simulink model "LUPAold"  (R2025b)
settings: Solver=FixedStepAuto  StartTime=0.0  StopTime=inf  FixedStep=Ts  RelTol=1e-3
PreLoadFcn:
  | addpath(genpath('utils'))
model workspace (MAT data in the model file):
  Sig = Simulink.Signal
  Sig.Dimensions = -1
  Sig.DimensionsMode = 'auto'
  Sig.Complexity = 'auto'
  Sig.SampleTime = -1
  Sig.SamplingMode = 'auto'
  Sig.DataType = 'auto'
values from neighbouring files (symbols this model uses):
  C = 258.803991051052    (= 258.803991051)    [AOE_constants.m]
  ExcelGains = table2array(ExcelGains)    [initLUPA.m]
  gainTstep = wavePeriod*10    (= 22.5)    [initLUPA.m]
  Kt = 7.86    [initLUPA.m]
  rampTime = 20    [initLUPA.m]
  sprocketPitchRadius = 0.101854    [initLUPA.m]
  Ts = 0.001    [initLUPA.m]
undefined symbols (not defined in the file or in its folder): drawWire_m, drawWire_mpers, eCATstate, linearPower_W, netForce_N, opState, pos_filt_rad, tet, vel_filt_radpers
libraries: slrealtimeethercatlib x26, slrealtimeloglib x12, simulink x6, dspfdesign x6, slrealtimeutilitieslib x4, dspstat3 x3, eeGeneralControl x3, slrealtimeptplib x1, slrealtimetgmanagement x1
settings Model: SimulationMode=external  ExtModeEnableFloating=off  Creator=HWRL user  LastModifiedBy=bosmab
settings SolverCC: ConcurrentTasks=on  PositivePriorityOrder=on
settings DataIOCC: ExternalInput=ds  LoadExternalInput=on
settings OptimizationCC: BlockReduction=off  OptimizeBlockIOStorage=off  ReuseModelBlockBuffer=off
settings DebuggingCC: TasksWithSamePriorityMsg=none  ParameterOverflowMsg=warning  ParameterPrecisionLossMsg=none  UnconnectedInputMsg=warning  UnconnectedOutputMsg=warning  UnconnectedLineMsg=warning
settings HardwareCC: ProdBitPerLong=64.0  ProdLongLongMode=on  ProdHWDeviceType=Intel->x86-64 (Linux 64)
settings ModelReferenceCC: EnableRefExpFcnMdlSchedulingChecks=on
settings SFSimCC: SimTargetLang=C++  SimDLTargetLibrary=mkl-dnn
settings RTWCC: SystemTargetFile=speedgoat.tlc  TemplateMakefile=slrealtime_default_tmf  RTWVerbose=off  Toolchain=Simulink Real-Time Toolchain  BuildConfiguration=Faster Runs  CodeExecutionProfiling=on  TargetLang=C++  GPUComputeCapability=3.5  DLArmComputeVersion=19.05  Description=Speedgoat Real-Time Target Machine
settings SimulinkRealTimeTargetCC: SLRTFileLogMaxRuns=1.0  ExtModeMaxTrigDuration=10.0  ExtModeStaticAllocSize=1000000.0  ExtModeTransport=0.0  MultiwordLength=2048.0  DynamicStringBufferSize=256.0  PreserveMATLABNamespacesInGeneratedCode=on  SubcomponentCodeInterfacePackaging=Reusable function  InstructionSetFMA=off  LogToMDFFile=off

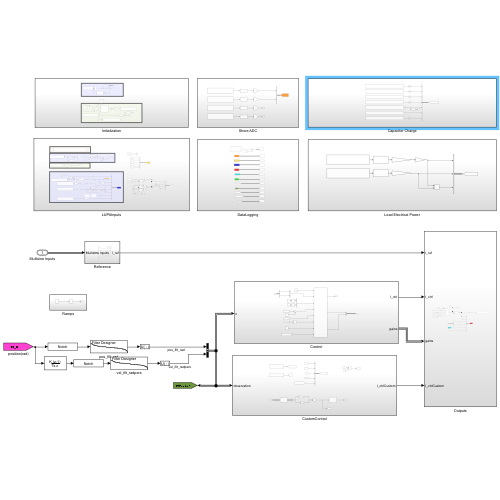
[thumbnail: Simulink's stored preview of the top-level diagram]
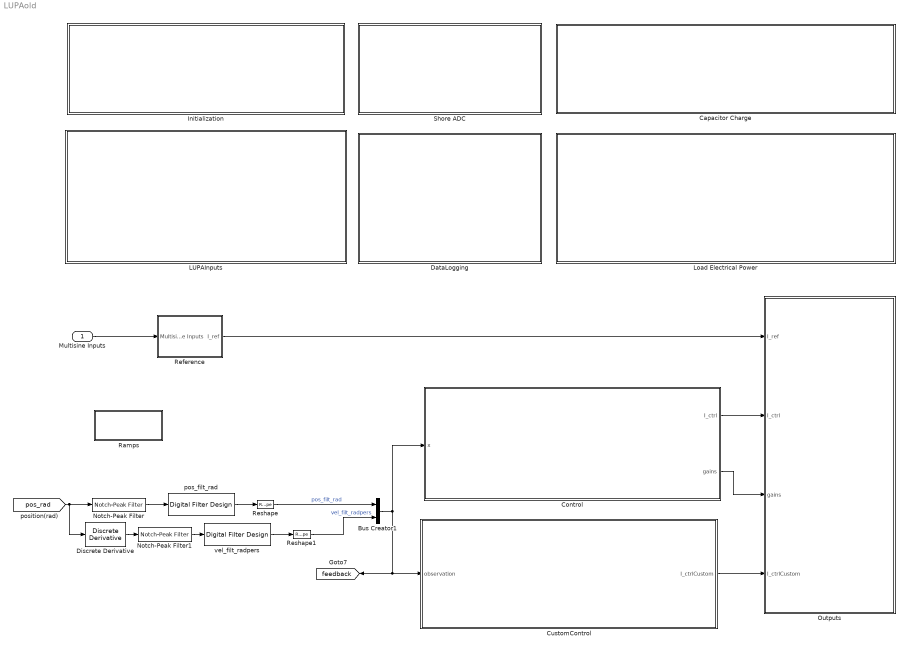
== system LUPAold ==
  Multisine Inputs : Inport  OutDataTypeStr=Bus: refSigs
  Bus Creator1 : BusCreator  Inputs=pos_filt_rad,vel_filt_radpers
  Capacitor Charge : Subsystem
  Control : Subsystem
  CustomControl : Subsystem
  DataLogging : Subsystem
  Discrete Derivative : simulink/Discrete/Discrete Derivative  gainval=1.0  ICPrevScaledInput=0.0  OutMin=[]  OutMax=[]  OutDataType=fixdt(1, 16)  OutScaling=2^-10  DoSatur=off
  Initialization : Subsystem
  LUPAInputs : Subsystem
  Load Electrical Power : Subsystem
  Notch-Peak Filter : dspfdesign/Notch-Peak Filter  Specification=Bandwidth and center frequency  BandwidthPort=off  Bandwidth=10  QualityFactorPort=off  QualityFactor=5  CenterFrequencyPort=off  CenterFrequency=50  BandwidthCoefficientPort=off  BandwidthCoefficient=0.72654  CenterFrequencyCoefficientPort=off  CenterFrequencyCoefficient=0  Output=Notch  SampleRateMode=Specify on dialog  SampleRate=1000  SimulateUsing=Code generation
  Notch-Peak Filter1 : dspfdesign/Notch-Peak Filter  Specification=Bandwidth and center frequency  BandwidthPort=off  Bandwidth=10  QualityFactorPort=off  QualityFactor=5  CenterFrequencyPort=off  CenterFrequency=50  BandwidthCoefficientPort=off  BandwidthCoefficient=0.72654  CenterFrequencyCoefficientPort=off  CenterFrequencyCoefficient=0  Output=Notch  SampleRateMode=Specify on dialog  SampleRate=1000  SimulateUsing=Code generation
  Outputs : Subsystem
  Ramps : Subsystem
  Reference : Subsystem
  Reshape : Reshape
  Reshape1 : Reshape
  Shore ADC : Subsystem
  pos_filt_rad : dspfdesign/Digital Filter Design  mwdsp_browser_bugfix_var=off
  vel_filt_radpers : dspfdesign/Digital Filter Design  mwdsp_browser_bugfix_var=off
  tag scope: feedback=global
  wires:
  Control/1(I_ctrl) -> Outputs/2(I_ctrl)
  Bus Creator1/1 -> Control/1(x), [feedback], CustomControl/1(observation)
  [pos_rad] -> Discrete Derivative/1, Notch-Peak Filter/1
  Control/2(gains) -> Outputs/3(gains)
  CustomControl/1(I_ctrlCustom) -> Outputs/4(I_ctrlCustom)
  Reference/1(I_ref) -> Outputs/1(I_ref)
  Multisine Inputs/1 -> Reference/1(Multisine Inputs)
  Notch-Peak Filter/1 -> pos_filt_rad/1
  Notch-Peak Filter1/1 -> vel_filt_radpers/1
  Discrete Derivative/1 -> Notch-Peak Filter1/1
  pos_filt_rad/1 -> Reshape/1
  vel_filt_radpers/1 -> Reshape1/1
  Reshape/1 -> Bus Creator1/1  "pos_filt_rad"
  Reshape1/1 -> Bus Creator1/2  "vel_filt_radpers"

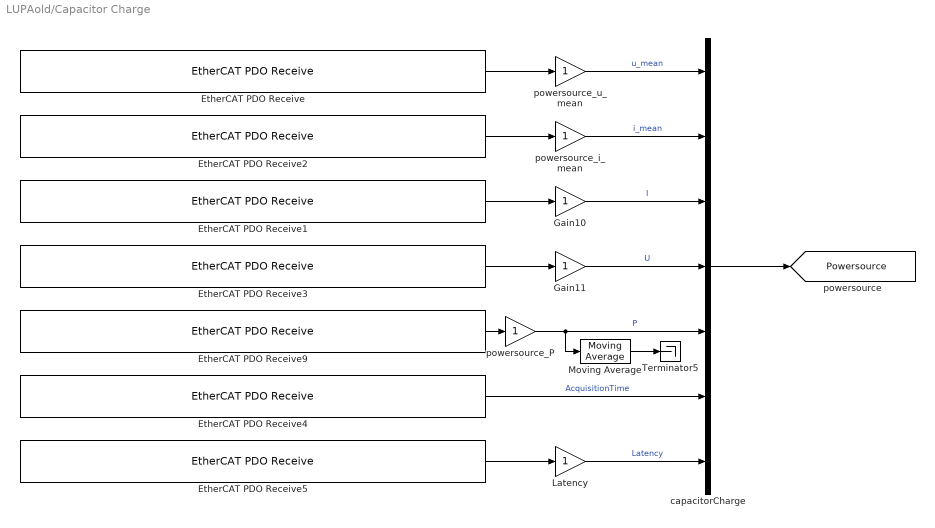
== system LUPAold/Capacitor Charge ==
  EtherCAT PDO Receive : slrealtimeethercatlib/EtherCAT PDO Receive  Priority=2  sig_name=Box 1 (GEN Series DAQ System).Powersource.out.u_mean.Powersource.out.u_mean_V  sig_offset=2648  sig_type=single  type_size=32  sig_dim=1  device_id=0  sample_time=0.001000
  EtherCAT PDO Receive1 : slrealtimeethercatlib/EtherCAT PDO Receive  Priority=2  sig_name=Box 1 (GEN Series DAQ System).Powersource.out.I.Powersource.out.I_V  sig_offset=2528  sig_type=single  type_size=32  sig_dim=1  device_id=0  sample_time=0.001000
  EtherCAT PDO Receive2 : slrealtimeethercatlib/EtherCAT PDO Receive  Priority=2  sig_name=Box 1 (GEN Series DAQ System).Powersource.out.i_mean.Powersource.out.i_mean_V  sig_offset=2608  sig_type=single  type_size=32  sig_dim=1  device_id=0  sample_time=0.001000
  EtherCAT PDO Receive3 : slrealtimeethercatlib/EtherCAT PDO Receive  Priority=2  sig_name=Box 1 (GEN Series DAQ System).Powersource.out.U.Powersource.out.U_V  sig_offset=2568  sig_type=single  type_size=32  sig_dim=1  device_id=0  sample_time=0.001000
  EtherCAT PDO Receive4 : slrealtimeethercatlib/EtherCAT PDO Receive  Priority=2  sig_name=Box 1 (GEN Series DAQ System).AcquisitionTime.AcquisitionTime_V  sig_offset=2296  sig_type=double  type_size=64  sig_dim=1  device_id=0  sample_time=0.001000
  EtherCAT PDO Receive5 : slrealtimeethercatlib/EtherCAT PDO Receive  Priority=2  sig_name=Box 1 (GEN Series DAQ System).Latency.Latency_V  sig_offset=2368  sig_type=single  type_size=32  sig_dim=1  device_id=0  sample_time=0.001000
  EtherCAT PDO Receive9 : slrealtimeethercatlib/EtherCAT PDO Receive  Priority=2  sig_name=Box 1 (GEN Series DAQ System).Powersource.out.P.Powersource.out.P_V  sig_offset=2688  sig_type=single  type_size=32  sig_dim=1  device_id=0  sample_time=0.001000
  Gain10 : Gain  OutDataTypeStr=double
  Gain11 : Gain  OutDataTypeStr=double
  Latency : Gain  OutDataTypeStr=double
  Moving Average : dspstat3/Moving Average  Method=Sliding window  ForgettingFactorPort=off  SpecifyWindowLength=on  WindowLength=10000  OverlapLength=9000  AllowArbitraryInputLength=on  ForgettingFactor=0.9  SimulateUsing=Code generation
  Terminator5 : Terminator
  capacitorCharge : BusCreator  Inputs=7
  powersource_P : Gain  OutDataTypeStr=double
  powersource_i_mean : Gain  OutDataTypeStr=double
  powersource_u_mean : Gain  OutDataTypeStr=double
  tag scope: Powersource=global
  wires:
  powersource_u_mean/1 -> capacitorCharge/1  "u_mean"
  powersource_i_mean/1 -> capacitorCharge/2  "i_mean"
  capacitorCharge/1 -> [Powersource]
  Gain10/1 -> capacitorCharge/3  "I"
  Gain11/1 -> capacitorCharge/4  "U"
  EtherCAT PDO Receive/1 -> powersource_u_mean/1
  EtherCAT PDO Receive2/1 -> powersource_i_mean/1
  EtherCAT PDO Receive1/1 -> Gain10/1
  EtherCAT PDO Receive3/1 -> Gain11/1
  EtherCAT PDO Receive9/1 -> powersource_P/1
  powersource_P/1 -> Moving Average/1, capacitorCharge/5  "P"
  EtherCAT PDO Receive4/1 -> capacitorCharge/6  "AcquisitionTime"
  EtherCAT PDO Receive5/1 -> Latency/1
  Latency/1 -> capacitorCharge/7  "Latency"
  Moving Average/1 -> Terminator5/1

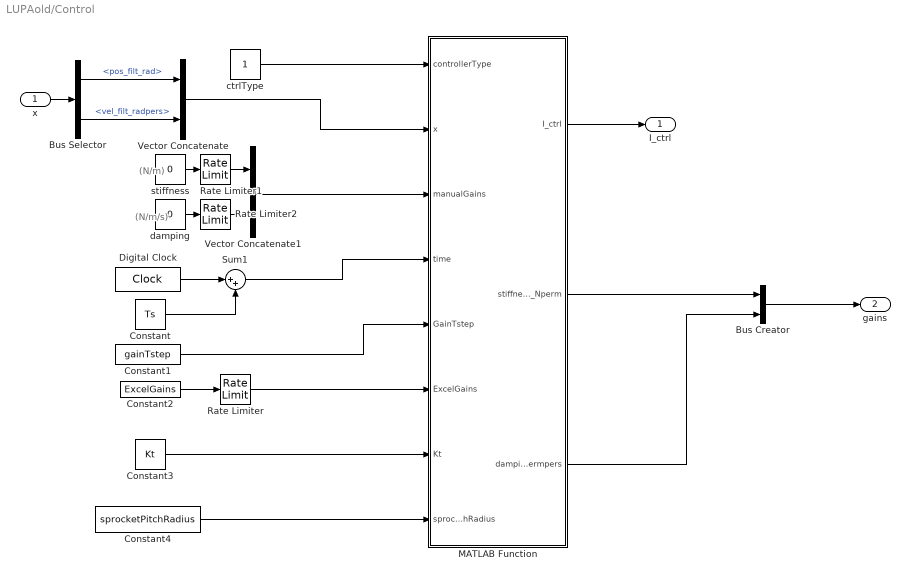
== system LUPAold/Control ==
  note: (N/m/s)
  note: (N/m)
  x : Inport
  Bus Creator : BusCreator  Inputs=2
  Bus Selector : BusSelector  OutputSignals=pos_filt_rad,vel_filt_radpers
  Constant : Constant  Value=Ts
  Constant1 : Constant  Value=gainTstep
  Constant2 : Constant  Value=ExcelGains  VectorParams1D=off
  Constant3 : Constant  Value=Kt
  Constant4 : Constant  Value=sprocketPitchRadius
  Digital Clock : DigitalClock  SampleTime=Ts
  MATLAB Function : MATLAB Function  TreatAsAtomicUnit=on
  Rate Limiter : RateLimiter  RisingSlewLimit=200  FallingSlewLimit=-200  SampleTimeMode=inherited
  Rate Limiter1 : RateLimiter  RisingSlewLimit=200  FallingSlewLimit=-200  SampleTimeMode=inherited
  Rate Limiter2 : RateLimiter  RisingSlewLimit=200  FallingSlewLimit=-200  SampleTimeMode=inherited
  Sum1 : Sum  Inputs=|++
  Vector Concatenate : Concatenate  Mode=Multidimensional array
  Vector Concatenate1 : Concatenate  Mode=Multidimensional array
  ctrlType : Constant
  damping : Constant  Value=0
  stiffness : Constant  Value=0
  I_ctrl : Outport
  gains : Outport  Port=2
  wires:
  stiffness/1 -> Rate Limiter1/1
  Constant1/1 -> MATLAB Function/5(GainTstep)
  Constant/1 -> Sum1/2
  Vector Concatenate1/1 -> MATLAB Function/3(manualGains)
  Digital Clock/1 -> Sum1/1
  x/1 -> Bus Selector/1
  Sum1/1 -> MATLAB Function/4(time)
  Constant4/1 -> MATLAB Function/8(sprocketPitchRadius)
  damping/1 -> Rate Limiter2/1
  Vector Concatenate/1 -> MATLAB Function/2(x)
  ctrlType/1 -> MATLAB Function/1(controllerType)
  Constant3/1 -> MATLAB Function/7(Kt)
  Constant2/1 -> Rate Limiter/1
  Bus Selector/1 -> Vector Concatenate/1  "<pos_filt_rad>"
  Bus Selector/2 -> Vector Concatenate/2  "<vel_filt_radpers>"
  MATLAB Function/1(I_ctrl) -> I_ctrl/1
  MATLAB Function/2(stiffness_Nperm) -> Bus Creator/1
  MATLAB Function/3(damping_Npermpers) -> Bus Creator/2
  Bus Creator/1 -> gains/1
  Rate Limiter/1 -> MATLAB Function/6(ExcelGains)
  Rate Limiter1/1 -> Vector Concatenate1/1
  Rate Limiter2/1 -> Vector Concatenate1/2

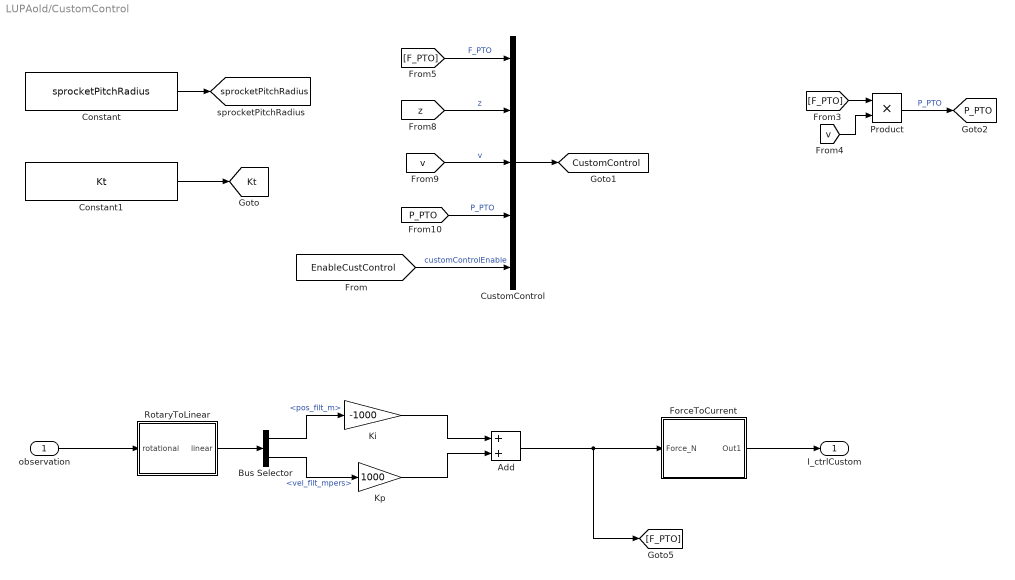
== system LUPAold/CustomControl ==
  observation : Inport
  Add : Sum
  Bus Selector : BusSelector  OutputSignals=pos_filt_m,vel_filt_mpers
  Constant : Constant  Value=sprocketPitchRadius
  Constant1 : Constant  Value=Kt
  CustomControl : BusCreator  Inputs=5
  ForceToCurrent : Subsystem
  Ki : Gain  Gain=-1000
  Kp : Gain  Gain=1000
  Product : Product
  RotaryToLinear : Subsystem
  I_ctrlCustom : Outport
  tag scope: CustomControl=global, Kt=global, P_PTO=global, sprocketPitchRadius=global
  wires:
  Constant/1 -> [sprocketPitchRadius]
  Constant1/1 -> [Kt]
  ForceToCurrent/1(Out1) -> I_ctrlCustom/1
  [F_PTO] -> Product/1
  [v] -> Product/2
  Product/1 -> [P_PTO]  "P_PTO"
  observation/1 -> RotaryToLinear/1(rotational)
  CustomControl/1 -> [CustomControl]
  [F_PTO] -> CustomControl/1  "F_PTO"
  [z] -> CustomControl/2  "z"
  [v] -> CustomControl/3  "v"
  [P_PTO] -> CustomControl/4  "P_PTO"
  RotaryToLinear/1(linear) -> Bus Selector/1
  Bus Selector/1 -> Ki/1  "<pos_filt_m>"
  Bus Selector/2 -> Kp/1  "<vel_filt_mpers>"
  Ki/1 -> Add/1
  Kp/1 -> Add/2
  Add/1 -> [F_PTO], ForceToCurrent/1(Force_N)
  [EnableCustControl] -> CustomControl/5  "customControlEnable"

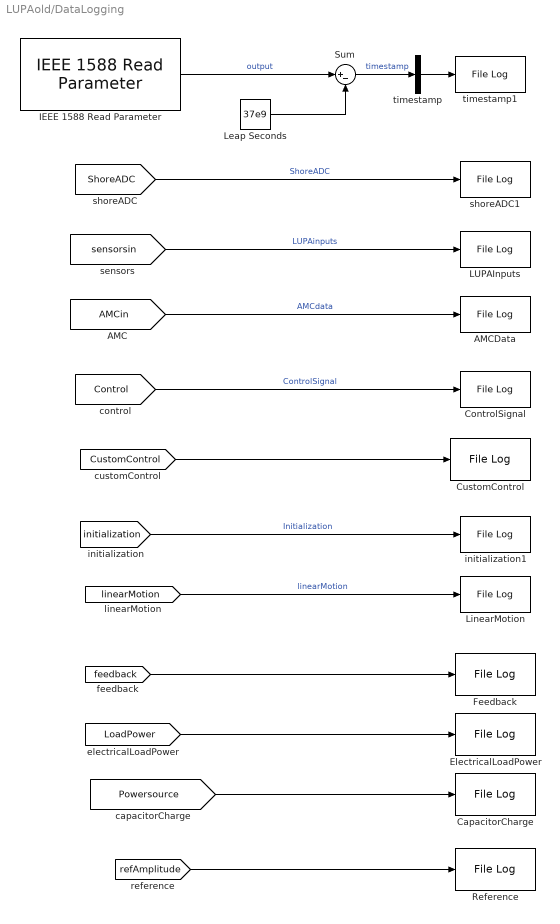
== system LUPAold/DataLogging ==
  AMCData : slrealtimeloglib/File Log  decimation=decimationLog  inputProcessing=Elements as channels (sample based)
  CapacitorCharge : slrealtimeloglib/File Log  decimation=1  inputProcessing=Elements as channels (sample based)
  ControlSignal : slrealtimeloglib/File Log  decimation=decimationLog  inputProcessing=Elements as channels (sample based)
  CustomControl : slrealtimeloglib/File Log  decimation=decimationLog  inputProcessing=Elements as channels (sample based)
  ElectricalLoadPower : slrealtimeloglib/File Log  decimation=1  inputProcessing=Elements as channels (sample based)
  Feedback : slrealtimeloglib/File Log  decimation=1  inputProcessing=Elements as channels (sample based)
  IEEE 1588 Read Parameter : slrealtimeptplib/IEEE 1588 Read Parameter  Priority=1  ID=1  param=1. System time (nanosecond)  sample_time=Ts
  LUPAInputs : slrealtimeloglib/File Log  decimation=decimationLog  inputProcessing=Elements as channels (sample based)
  Leap Seconds : Constant  Value=37e9  OutDataTypeStr=double
  LinearMotion : slrealtimeloglib/File Log  decimation=decimationLog  inputProcessing=Elements as channels (sample based)
  Reference : slrealtimeloglib/File Log  decimation=1  inputProcessing=Elements as channels (sample based)
  Sum : Sum  Inputs=|+-
  initialization1 : slrealtimeloglib/File Log  decimation=decimationLog  inputProcessing=Elements as channels (sample based)
  shoreADC1 : slrealtimeloglib/File Log  decimation=decimationLog  inputProcessing=Elements as channels (sample based)
  timestamp : BusCreator  Inputs=timestamp
  timestamp1 : slrealtimeloglib/File Log  decimation=decimationLog  inputProcessing=Elements as channels (sample based)
  wires:
  [AMCin] -> AMCData/1  "AMCdata"
  [Control] -> ControlSignal/1  "ControlSignal"
  IEEE 1588 Read Parameter/1 -> Sum/1  "output"
  Sum/1 -> timestamp/1  "timestamp"
  timestamp/1 -> timestamp1/1
  Leap Seconds/1 -> Sum/2
  [initialization] -> initialization1/1  "Initialization"
  [sensorsin] -> LUPAInputs/1  "LUPAinputs"
  [ShoreADC] -> shoreADC1/1  "ShoreADC"
  [linearMotion] -> LinearMotion/1  "linearMotion"
  [feedback] -> Feedback/1
  [CustomControl] -> CustomControl/1
  [LoadPower] -> ElectricalLoadPower/1
  [Powersource] -> CapacitorCharge/1
  [refAmplitude] -> Reference/1

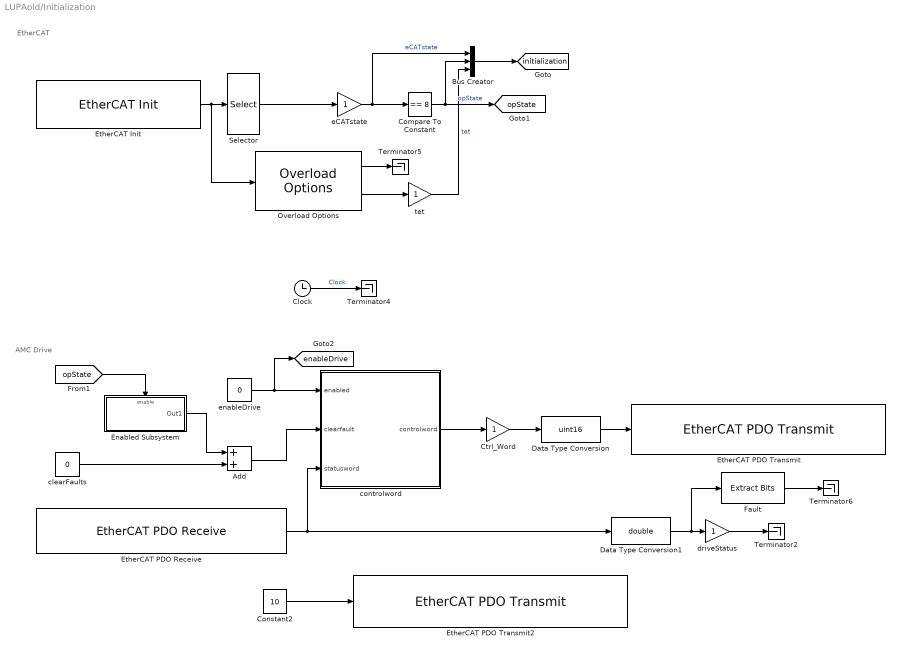
== system LUPAold/Initialization ==
  note: AMC Drive
  note: EtherCAT
  Add : Sum
  Bus Creator : BusCreator  Inputs=eCATstate,opState,tet
  Clock : Clock
  Compare To Constant : simulink/Logic and Bit Operations/Compare To Constant  relop===  const=8  OutDataTypeStr=boolean
  Constant2 : Constant  Value=10  OutDataTypeStr=uint16
  Ctrl_Word : Gain
  Data Type Conversion : DataTypeConversion  OutDataTypeStr=uint16  SaturateOnIntegerOverflow=off  RndMeth=Floor
  Data Type Conversion1 : DataTypeConversion  OutDataTypeStr=double  SaturateOnIntegerOverflow=off  RndMeth=Floor
  Enabled Subsystem : Subsystem  TreatAsAtomicUnit=on
  EtherCAT Init : slrealtimeethercatlib/EtherCAT Init  Priority=0  config_file=C:\Software\LUPA\Simulink\EtherCAT\LUPAxml.xml  device_id=0  portnum=1  initstate=2  dctuning=0  enaDebug=0  logFile='c:\dbglog.txt'  sample_time=0.001000  DCMode=2
  EtherCAT PDO Receive : slrealtimeethercatlib/EtherCAT PDO Receive  Priority=2  sig_name=Drive 7 (AMC - DPE X2.1).PDO data from Slave.Status Word  sig_offset=576  sig_type=uint16  type_size=16  sig_dim=1  device_id=0  sample_time=0.001000
  EtherCAT PDO Transmit : slrealtimeethercatlib/EtherCAT PDO Transmit  Priority=3  sig_name=Drive 7 (AMC - DPE X2.1).PDO data to Slave.Control Word  sig_offset=576  sig_type=uint16  type_size=16  sig_dim=1  device_id=0  sample_time=0.001000
  EtherCAT PDO Transmit2 : slrealtimeethercatlib/EtherCAT PDO Transmit  Priority=3  sig_name=Drive 7 (AMC - DPE X2.1).PDO data to Slave.Modes Of Operation  sig_offset=688  sig_type=uint16  type_size=16  sig_dim=1  device_id=0  sample_time=0.001000
  Fault : simulink/Logic and Bit Operations/Extract Bits  bitsToExtract=Range of bits  numBits=8  bitIdxRange=[3]  outScalingMode=Preserve fixed-point scaling
  Overload Options : slrealtimetgmanagement/Overload Options  startupDur=1  startupDurSrc=Tunable Parameter  maxOverload=0  maxOverloadSrc=Tunable Parameter  TETFlag=on
  Selector : Selector  InputPortWidth=6  IndexOptions=Index vector (dialog)  Indices=2  OutputSizes=1
  Terminator{2,4..6} (4 alike) : Terminator
  clearFaults : Constant  Value=0
  controlword : MATLAB Function  TreatAsAtomicUnit=on
  driveStatus : Gain
  eCATstate : Gain  OutDataTypeStr=double
  enableDrive : Constant  Value=0
  tet : Gain  OutDataTypeStr=double
  tag scope: enableDrive=global, initialization=global, opState=global
  wires:
  EtherCAT Init/1 -> Overload Options/1, Selector/1
  Selector/1 -> eCATstate/1
  Compare To Constant/1 -> [opState], Bus Creator/2  "opState"
  EtherCAT PDO Receive/1 -> Data Type Conversion1/1, controlword/3(statusword)
  Constant2/1 -> EtherCAT PDO Transmit2/1
  Data Type Conversion1/1 -> Fault/1, driveStatus/1
  controlword/1(controlword) -> Ctrl_Word/1
  Data Type Conversion/1 -> EtherCAT PDO Transmit/1
  driveStatus/1 -> Terminator2/1
  Ctrl_Word/1 -> Data Type Conversion/1
  enableDrive/1 -> [enableDrive], controlword/1(enabled)
  eCATstate/1 -> Bus Creator/1, Compare To Constant/1  "eCATstate"
  Clock/1 -> Terminator4/1  "Clock"
  Bus Creator/1 -> [initialization]
  Overload Options/2 -> tet/1
  tet/1 -> Bus Creator/3  "tet"
  Overload Options/1 -> Terminator5/1
  Fault/1 -> Terminator6/1
  Enabled Subsystem/1(Out1) -> Add/1
  [opState] -> Enabled Subsystem/Enable
  Add/1 -> controlword/2(clearfault)
  clearFaults/1 -> Add/2

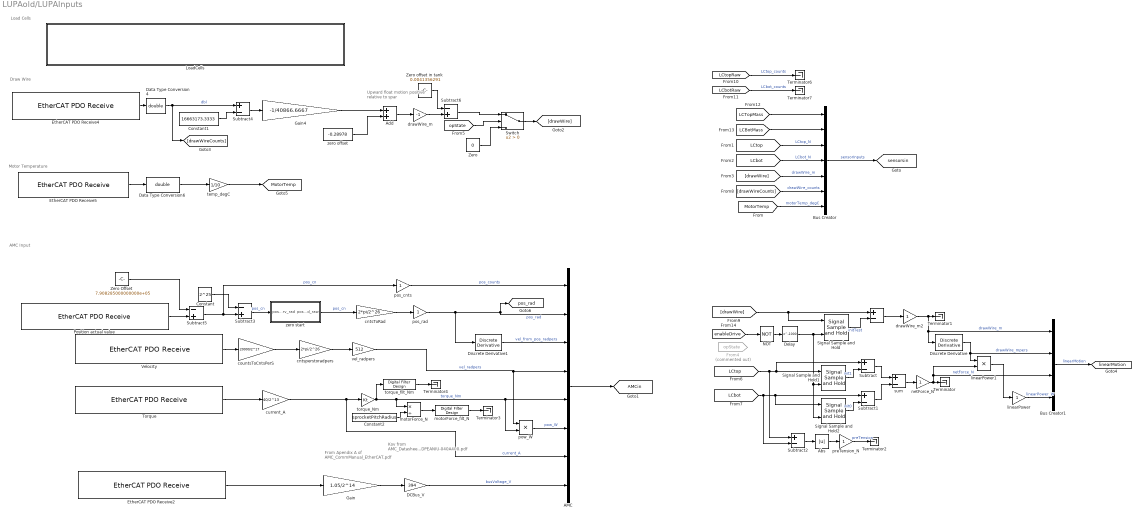
== system LUPAold/LUPAInputs ==
  note: Load Cells
  note: Upward float motion
      | positive relative to spar
  note: Draw Wire
  note: Motor Temperature
  note: From Apendix A of AMC_CommManual_EtherCAT.pdf
  note: AMC Input
  note: Kov from AMC_Datasheet_DPEANIU-040A400.pdf
  " " : Sum  Inputs=+-
  AMC : BusCreator  Inputs=8
  Abs : Abs  SaturateOnIntegerOverflow=off
  Add : Sum
  Bus Creator : BusCreator  Inputs=7
  Bus Creator1 : BusCreator  Inputs=drawWire_m,drawWire_mpers,netForce_N,linearPower_W
  Constant : Constant  Value=2^25
  Constant1 : Constant  Value=16663173.3333
  Constant2 : Constant  Value=sprocketPitchRadius
  DCBus_V : Gain  Gain=394
  Data Type Conversion4 : DataTypeConversion  OutDataTypeStr=double  SaturateOnIntegerOverflow=off  RndMeth=Floor
  Data Type Conversion6 : DataTypeConversion  OutDataTypeStr=double  SaturateOnIntegerOverflow=off  RndMeth=Floor
  Delay : Delay  DelayLength=1000
  Discrete Derivative : simulink/Discrete/Discrete Derivative  gainval=1.0  ICPrevScaledInput=0.0  OutMin=[]  OutMax=[]  OutDataType=fixdt(1, 16)  OutScaling=2^-10  DoSatur=off
  Discrete Derivative1 : simulink/Discrete/Discrete Derivative  gainval=1.0  ICPrevScaledInput=0.0  OutMin=[]  OutMax=[]  OutDataType=fixdt(1, 16)  OutScaling=2^-10  DoSatur=off
  EtherCAT PDO Receive2 : slrealtimeethercatlib/EtherCAT PDO Receive  Priority=2  sig_name=Drive 7 (AMC - DPE X2.1).PDO data from Slave.DC Bus Voltage  sig_offset=688  sig_type=uint16  type_size=16  sig_dim=1  device_id=0  sample_time=0.001000
  EtherCAT PDO Receive4 : slrealtimeethercatlib/EtherCAT PDO Receive  Priority=2  sig_name=Term 9 (EL5002).SSI Inputs Channel 1.Counter value  sig_offset=1216  sig_type=uint32  type_size=32  sig_dim=1  device_id=0  sample_time=0.001000
  EtherCAT PDO Receive5 : slrealtimeethercatlib/EtherCAT PDO Receive  Priority=2  sig_name=Term 12 (EL3202).RTD Inputs Channel 1.Value  sig_offset=2144  sig_type=int16  type_size=16  sig_dim=1  device_id=0  sample_time=0.001000
  From4 : From  Commented=on  GotoTag=opState  TagVisibility=global
  Gain : Gain  Gain=1.05/2^14  OutDataTypeStr=double
  Gain4 : Gain  Gain=-1/40866.6667
  LoadCells : Subsystem
  NOT : Logic  Operator=NOT  IconShape=distinctive  AllPortsSameDT=off  OutDataTypeStr=boolean
  Position actual value : slrealtimeethercatlib/EtherCAT PDO Receive  Priority=2  sig_name=Drive 7 (AMC - DPE X2.1).PDO data from Slave.Actual position  sig_offset=592  sig_type=int32  type_size=32  sig_dim=1  device_id=0  sample_time=0.001000
  Signal Sample and Hold : eeGeneralControl/Signal Sample and Hold  LabelModeActiveChoice=Discrete  x0=0  Ts=Ts
      settings: LibrarySourceBlock=ee_sl_lib/General Control/Signal Sample and Hold
  Signal Sample and Hold1 : eeGeneralControl/Signal Sample and Hold  LabelModeActiveChoice=Discrete  x0=0  Ts=Ts
      settings: LibrarySourceBlock=ee_sl_lib/General Control/Signal Sample and Hold
  Signal Sample and Hold2 : eeGeneralControl/Signal Sample and Hold  LabelModeActiveChoice=Discrete  x0=0  Ts=Ts
      settings: LibrarySourceBlock=ee_sl_lib/General Control/Signal Sample and Hold
  Subtract{,1..2,4} (4 alike) : Sum  Inputs=+-
  Subtract3 : Sum  Inputs=-+
  Subtract5 : Sum  Inputs=-+  OutDataTypeStr=double
  Subtract6 : Sum  Inputs=-+
  Switch : Switch  Criteria=u2 > Threshold  SaturateOnIntegerOverflow=off  InputSameDT=off
  Terminator{,1..4,6..7} (7 alike) : Terminator
  Torque : slrealtimeethercatlib/EtherCAT PDO Receive  Priority=2  sig_name=Drive 7 (AMC - DPE X2.1).PDO data from Slave.Actual Current  sig_offset=656  sig_type=int16  type_size=16  sig_dim=1  device_id=0  sample_time=0.001000
  Velocity : slrealtimeethercatlib/EtherCAT PDO Receive  Priority=2  sig_name=Drive 7 (AMC - DPE X2.1).PDO data from Slave.Actual Velocity  sig_offset=624  sig_type=int32  type_size=32  sig_dim=1  device_id=0  sample_time=0.001000
  Zero : Constant  Value=0  OutDataTypeStr=double
  Zero Offset : Constant  Value=7.908285000000000e+05
  Zero offset in tank : Constant  Value=0.0041356291
  cntsToRad : Gain  Gain=2*pi/2^26  OutDataTypeStr=double
  cntsperstoradpers : Gain  Gain=2*pi/2^26
  countsToCntsPerS : Gain  Gain=20000/2^17  OutDataTypeStr=double
  current_A : Gain  Gain=40/2^13  OutDataTypeStr=double
  drawWire_m : Gain  Gain=-1
  drawWire_m2 : Gain
  linearPower : Gain
  linearPower1 : Product
  motorForce_N : Product  Inputs=*/
  motorForce_filt_N : dspfdesign/Digital Filter Design  mwdsp_browser_bugfix_var=off
  netForce_N : Gain
  pos_cnts : Gain
  pos_rad : Gain
  pow_W : Product
  preTension_N : Gain
  sum : Sum  Inputs=+-
  temp_degC : Gain  Gain=1/10
  torque_Nm : Gain  Gain=Kt
  torque_filt_Nm : dspfdesign/Digital Filter Design  mwdsp_browser_bugfix_var=off
  vel_radpers : Gain  Gain=512
  zero offset : Constant  Value=-0.28978
  zero start : Subsystem
  tag scope: AMCin=global, MotorTemp=global, linearMotion=global, pos_rad=global, sensorsin=global
  wires:
  [opState] -> Switch/2
  drawWire_m/1 -> Subtract6/2
  EtherCAT PDO Receive4/1 -> Data Type Conversion4/1
  Switch/1 -> [drawWire]
  Data Type Conversion4/1 -> Subtract4/1, [drawWireCounts]  "dbl"
  Subtract4/1 -> Gain4/1
  Zero/1 -> Switch/3
  temp_degC/1 -> [MotorTemp]
  Data Type Conversion6/1 -> temp_degC/1
  EtherCAT PDO Receive5/1 -> Data Type Conversion6/1
  Bus Creator/1 -> [sensorsin]  "sensorInputs"
  [drawWire] -> Bus Creator/5  "drawWire_m"
  [LCtop] -> Bus Creator/3  "LCtop_N"
  [MotorTemp] -> Bus Creator/7  "motorTemp_degC"
  [LCbot] -> Bus Creator/4  "LCbot_N"
  torque_Nm/1 -> torque_filt_Nm/1, pow_W/2, AMC/5, motorForce_N/1  "torque_Nm"
  Discrete Derivative1/1 -> AMC/3  "vel_from_pos_radpers"
  Gain/1 -> DCBus_V/1
  vel_radpers/1 -> pow_W/1, AMC/4  "vel_radpers"
  pos_rad/1 -> Discrete Derivative1/1, [pos_rad], AMC/2  "pos_rad"
  Velocity/1 -> countsToCntsPerS/1
  Torque/1 -> current_A/1
  AMC/1 -> [AMCin]
  DCBus_V/1 -> AMC/8  "busVoltage_V"
  EtherCAT PDO Receive2/1 -> Gain/1
  Constant/1 -> Subtract3/1
  Subtract5/1 -> pos_cnts/1, Subtract3/2  "pos_cn"
  current_A/1 -> torque_Nm/1, AMC/7  "current_A"
  pow_W/1 -> AMC/6  "pow_W"
  cntsToRad/1 -> pos_rad/1
  [drawWire] -> Signal Sample and Hold/1, " "/1
  drawWire_m2/1 -> Bus Creator1/1, Discrete Derivative/1, Terminator1/1  "drawWire_m"
  netForce_N/1 -> Bus Creator1/3, linearPower1/2, Terminator/1  "netForce_N"
  sum/1 -> netForce_N/1
  Abs/1 -> preTension_N/1
  Subtract/1 -> sum/1
  Subtract2/1 -> Abs/1
  Signal Sample and Hold2/1 -> Subtract1/2  "init0"
  " "/1 -> drawWire_m2/1
  Discrete Derivative/1 -> Bus Creator1/2, linearPower1/1  "drawWire_mpers"
  Subtract1/1 -> sum/2
  preTension_N/1 -> Terminator2/1  "preTension"
  linearPower/1 -> Bus Creator1/4  "linearPower_W"
  Bus Creator1/1 -> [linearMotion]  "linearMotion"
  [LCbot] -> Subtract2/2, Signal Sample and Hold2/1, Subtract1/1
  linearPower1/1 -> linearPower/1
  Signal Sample and Hold1/1 -> Subtract/2  "init1"
  NOT/1 -> Delay/1
  Signal Sample and Hold/1 -> " "/2  "initTest"
  [LCtop] -> Subtract2/1, Subtract/1, Signal Sample and Hold1/1
  pos_cnts/1 -> AMC/1  "pos_counts"
  [LCtopRaw] -> Terminator6/1  "LCtop_counts"
  [LCbotRaw] -> Terminator7/1  "LCbot_counts"
  [LCTopMass] -> Bus Creator/1
  [LCBotMass] -> Bus Creator/2
  Position actual value/1 -> Subtract5/2
  Subtract3/1 -> zero start/1(pos_drv_rad)  "pos_cn"
  cntsperstoradpers/1 -> vel_radpers/1
  countsToCntsPerS/1 -> cntsperstoradpers/1
  zero start/1(pos_rad_raw) -> cntsToRad/1  "pos_cn"
  [drawWireCounts] -> Bus Creator/6  "drawWire_counts"
  Constant1/1 -> Subtract4/2
  Add/1 -> drawWire_m/1
  Gain4/1 -> Add/1
  zero offset/1 -> Add/2
  [enableDrive] -> NOT/1
  Delay/1 -> Signal Sample and Hold/2, Signal Sample and Hold1/2, Signal Sample and Hold2/2
  Constant2/1 -> motorForce_N/2
  motorForce_N/1 -> motorForce_filt_N/1
  motorForce_filt_N/1 -> Terminator3/1
  torque_filt_Nm/1 -> Terminator4/1
  Zero Offset/1 -> Subtract5/1
  Subtract6/1 -> Switch/1
  Zero offset in tank/1 -> Subtract6/1

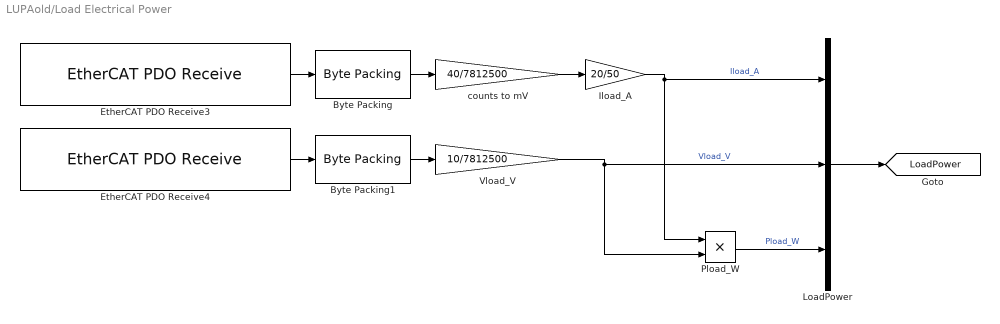
== system LUPAold/Load Electrical Power ==
  Byte Packing : slrealtimeutilitieslib/Byte Packing  MaskPackedDataType=int32  MaskUnpackedDataTypes={'uint8'}  MaskAlignment=1
  Byte Packing1 : slrealtimeutilitieslib/Byte Packing  MaskPackedDataType=int32  MaskUnpackedDataTypes={'uint8'}  MaskAlignment=1
  EtherCAT PDO Receive3 : slrealtimeethercatlib/EtherCAT PDO Receive  Priority=2  sig_name=Term 3 (EL3751).PAI Samples 1.Samples  sig_offset=848  sig_type=uint8  type_size=8  sig_dim=4  device_id=0  sample_time=0.001000
  EtherCAT PDO Receive4 : slrealtimeethercatlib/EtherCAT PDO Receive  Priority=2  sig_name=Term 4 (EL3751).PAI Samples 1.Samples  sig_offset=976  sig_type=uint8  type_size=8  sig_dim=4  device_id=0  sample_time=0.001000
  Iload_A : Gain  Gain=20/50
  LoadPower : BusCreator  Inputs=3
  Pload_W : Product
  Vload_V : Gain  Gain=10/7812500  OutDataTypeStr=double
  counts to mV : Gain  Gain=40/7812500  OutDataTypeStr=double
  tag scope: LoadPower=global
  wires:
  Byte Packing/1 -> counts to mV/1
  EtherCAT PDO Receive4/1 -> Byte Packing1/1
  EtherCAT PDO Receive3/1 -> Byte Packing/1
  Pload_W/1 -> LoadPower/3  "Pload_W"
  Byte Packing1/1 -> Vload_V/1
  Vload_V/1 -> Pload_W/2, LoadPower/2  "Vload_V"
  Iload_A/1 -> Pload_W/1, LoadPower/1  "Iload_A"
  counts to mV/1 -> Iload_A/1
  LoadPower/1 -> [LoadPower]

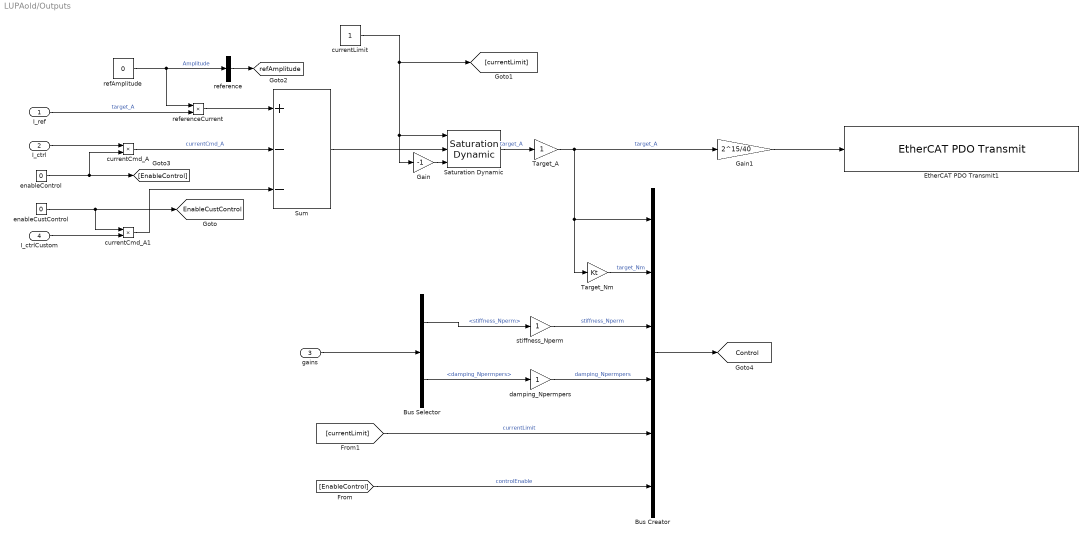
== system LUPAold/Outputs ==
  I_ref : Inport
  I_ctrl : Inport  Port=2
  gains : Inport  Port=3
  I_ctrlCustom : Inport  Port=4
  Bus Creator : BusCreator  Inputs=6
  Bus Selector : BusSelector  OutputSignals=stiffness_Nperm,damping_Npermpers
  EtherCAT PDO Transmit1 : slrealtimeethercatlib/EtherCAT PDO Transmit  Priority=3  sig_name=Drive 7 (AMC - DPE X2.1).PDO data to Slave.Target Current  sig_offset=656  sig_type=int16  type_size=16  sig_dim=1  device_id=0  sample_time=0.001000
  Gain : Gain  Gain=-1
  Gain1 : Gain  Gain=2^15/40  OutDataTypeStr=int16
  Saturation Dynamic : simulink/Discontinuities/Saturation Dynamic  OutMin=[]  OutMax=[]  OutDataTypeStr=Inherit: Same as second input  OutDataType=fixdt(1, 16)  OutScaling=2^-10  DoSatur=off
  Sum : Sum  Inputs=+--
  Target_A : Gain
  Target_Nm : Gain  Gain=Kt
  currentCmd_A : Product
  currentCmd_A1 : Product
  currentLimit : Constant
  damping_Npermpers : Gain
  enableControl : Constant  Value=0
  enableCustControl : Constant  Value=0
  refAmplitude : Constant  Value=0
  reference : BusCreator  Inputs=1
  referenceCurrent : Product
  stiffness_Nperm : Gain
  tag scope: Control=global, EnableCustControl=global, refAmplitude=global
  wires:
  Gain1/1 -> EtherCAT PDO Transmit1/1
  currentCmd_A/1 -> Sum/2  "currentCmd_A"
  currentLimit/1 -> Saturation Dynamic/1, Gain/1, [currentLimit]
  enableControl/1 -> [EnableControl], currentCmd_A/2
  I_ctrl/1 -> currentCmd_A/1
  Gain/1 -> Saturation Dynamic/3
  Saturation Dynamic/1 -> Target_A/1  "target_A"
  Bus Selector/2 -> damping_Npermpers/1  "<damping_Npermpers>"
  Target_Nm/1 -> Bus Creator/2  "target_Nm"
  Bus Selector/1 -> stiffness_Nperm/1  "<stiffness_Nperm>"
  stiffness_Nperm/1 -> Bus Creator/3  "stiffness_Nperm"
  Bus Creator/1 -> [Control]
  damping_Npermpers/1 -> Bus Creator/4  "damping_Npermpers"
  gains/1 -> Bus Selector/1
  currentCmd_A1/1 -> Sum/3
  I_ctrlCustom/1 -> currentCmd_A1/2
  enableCustControl/1 -> [EnableCustControl], currentCmd_A1/1
  [currentLimit] -> Bus Creator/5  "currentLimit"
  Sum/1 -> Saturation Dynamic/2
  I_ref/1 -> referenceCurrent/2  "target_A"
  Target_A/1 -> Gain1/1, Target_Nm/1, Bus Creator/1  "target_A"
  referenceCurrent/1 -> Sum/1
  refAmplitude/1 -> reference/1, referenceCurrent/1  "Amplitude"
  reference/1 -> [refAmplitude]
  [EnableControl] -> Bus Creator/6  "controlEnable"

== system LUPAold/Ramps ==
  EnableRamps : Constant  Value=0  OutDataTypeStr=double
  Rate Limiter : RateLimiter  RisingSlewLimit=1/rampTime  FallingSlewLimit=-1/rampTime  SampleTimeMode=inherited
  Terminator : Terminator
  wires:
  EnableRamps/1 -> Rate Limiter/1
  Rate Limiter/1 -> Terminator/1

== system LUPAold/Reference ==
  Multisine Inputs : Inport
  Bus Selector : BusSelector  OutputSignals=MS1,MS2,MS3
  Bus Selector1 : BusSelector  OutputSignals=ramps,sine,chirp,BLWN
  Multiport Switch : MultiPortSwitch  Inputs=8  SaturateOnIntegerOverflow=off  InputSameDT=off
  None : Constant  Value=0
  Subsystem Reference : Subsystem  ReferencedSubsystem=referenceSigs
  inputSwitch : Constant
  I_ref : Outport
  wires:
  inputSwitch/1 -> Multiport Switch/1
  Bus Selector/3 -> Multiport Switch/7  "<MS3>"
  Subsystem Reference/1 -> Bus Selector1/1
  Bus Selector/2 -> Multiport Switch/6  "<MS2>"
  Bus Selector1/2 -> Multiport Switch/4  "<sine>"
  Bus Selector1/4 -> Multiport Switch/9  "<BLWN>"
  Bus Selector1/3 -> Multiport Switch/8  "<chirp>"
  None/1 -> Multiport Switch/2
  Bus Selector/1 -> Multiport Switch/5  "<MS1>"
  Bus Selector1/1 -> Multiport Switch/3  "<ramps>"
  Multiport Switch/1 -> I_ref/1  "I_ref"
  Multisine Inputs/1 -> Bus Selector/1

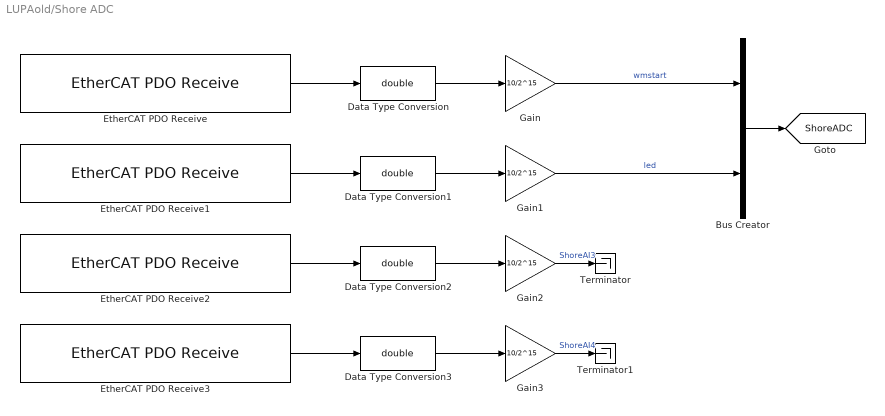
== system LUPAold/Shore ADC ==
  Bus Creator : BusCreator  Inputs=2
  Data Type Conversion{,1..3} (4 alike) : DataTypeConversion  OutDataTypeStr=double  SaturateOnIntegerOverflow=off  RndMeth=Floor
  EtherCAT PDO Receive : slrealtimeethercatlib/EtherCAT PDO Receive  Priority=2  sig_name=Term 6 (EL3104).AI Standard Channel 1.Value  sig_offset=1088  sig_type=int16  type_size=16  sig_dim=1  device_id=0  sample_time=0.001000
  EtherCAT PDO Receive1 : slrealtimeethercatlib/EtherCAT PDO Receive  Priority=2  sig_name=Term 6 (EL3104).AI Standard Channel 2.Value  sig_offset=1120  sig_type=int16  type_size=16  sig_dim=1  device_id=0  sample_time=0.001000
  EtherCAT PDO Receive2 : slrealtimeethercatlib/EtherCAT PDO Receive  Priority=2  sig_name=Term 6 (EL3104).AI Standard Channel 3.Value  sig_offset=1152  sig_type=int16  type_size=16  sig_dim=1  device_id=0  sample_time=0.001000
  EtherCAT PDO Receive3 : slrealtimeethercatlib/EtherCAT PDO Receive  Priority=2  sig_name=Term 6 (EL3104).AI Standard Channel 4.Value  sig_offset=1184  sig_type=int16  type_size=16  sig_dim=1  device_id=0  sample_time=0.001000
  Gain{,1..3} (4 alike) : Gain  Gain=10/2^15
  Terminator : Terminator
  Terminator1 : Terminator
  tag scope: ShoreADC=global
  wires:
  EtherCAT PDO Receive/1 -> Data Type Conversion/1
  EtherCAT PDO Receive1/1 -> Data Type Conversion1/1
  EtherCAT PDO Receive2/1 -> Data Type Conversion2/1
  EtherCAT PDO Receive3/1 -> Data Type Conversion3/1
  Bus Creator/1 -> [ShoreADC]
  Data Type Conversion/1 -> Gain/1
  Data Type Conversion1/1 -> Gain1/1
  Data Type Conversion2/1 -> Gain2/1
  Data Type Conversion3/1 -> Gain3/1
  Gain/1 -> Bus Creator/1  "wmstart"
  Gain3/1 -> Terminator1/1  "ShoreAI4"
  Gain2/1 -> Terminator/1  "ShoreAI3"
  Gain1/1 -> Bus Creator/2  "led"

== system LUPAold/CustomControl/ForceToCurrent ==
  Force_N : Inport
  Divide : Product  Inputs=*/
  Product : Product
  Out1 : Outport
  wires:
  [sprocketPitchRadius] -> Product/2
  Product/1 -> Divide/1  "torque_Nm"
  Divide/1 -> Out1/1
  Force_N/1 -> Product/1
  [Kt] -> Divide/2

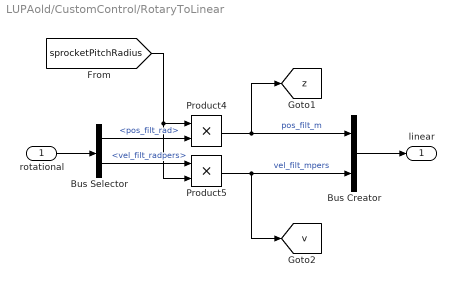
== system LUPAold/CustomControl/RotaryToLinear ==
  rotational : Inport
  Bus Creator : BusCreator  Inputs=2
  Bus Selector : BusSelector  OutputSignals=pos_filt_rad,vel_filt_radpers
  Product4 : Product
  Product5 : Product
  linear : Outport
  tag scope: v=global, z=global
  wires:
  Product5/1 -> [v], Bus Creator/2  "vel_filt_mpers"
  Bus Selector/1 -> Product4/2  "<pos_filt_rad>"
  Bus Creator/1 -> linear/1
  rotational/1 -> Bus Selector/1
  Product4/1 -> Bus Creator/1, [z]  "pos_filt_m"
  [sprocketPitchRadius] -> Product5/2, Product4/1
  Bus Selector/2 -> Product5/1  "<vel_filt_radpers>"

== system LUPAold/Initialization/Enabled Subsystem ==
  Enable : EnablePort
  Delay : Delay  DelayLength=1/Ts
  One : Constant  OutDataTypeStr=Inherit: Inherit via back propagation
  One1 : Constant  Value=-1  OutDataTypeStr=Inherit: Inherit via back propagation
  Sum : Sum  Inputs=|++
  Out1 : Outport
  wires:
  Sum/1 -> Out1/1
  One/1 -> Sum/1
  One1/1 -> Delay/1
  Delay/1 -> Sum/2

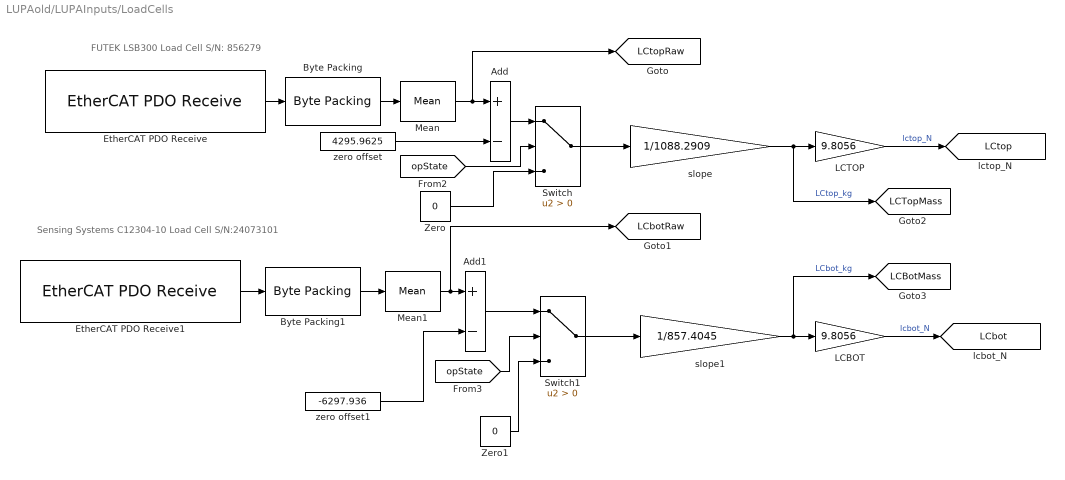
== system LUPAold/LUPAInputs/LoadCells ==
  note: FUTEK LSB300 Load Cell S/N: 856279
  note: Sensing Systems C12304-10 Load Cell S/N:24073101
  Add : Sum  Inputs=+-
  Add1 : Sum  Inputs=+-
  Byte Packing : slrealtimeutilitieslib/Byte Packing  MaskPackedDataType=int32  MaskUnpackedDataTypes={'uint8'}  MaskAlignment=1
  Byte Packing1 : slrealtimeutilitieslib/Byte Packing  MaskPackedDataType=int32  MaskUnpackedDataTypes={'uint8'}  MaskAlignment=1
  EtherCAT PDO Receive : slrealtimeethercatlib/EtherCAT PDO Receive  Priority=2  sig_name=Term 11 (EL3751).PAI Samples 10.Samples  sig_offset=1744  sig_type=uint8  type_size=8  sig_dim=40  device_id=0  sample_time=0.001000
  EtherCAT PDO Receive1 : slrealtimeethercatlib/EtherCAT PDO Receive  Priority=2  sig_name=Term 10 (EL3751).PAI Samples 10.Samples  sig_offset=1328  sig_type=uint8  type_size=8  sig_dim=40  device_id=0  sample_time=0.001000
  LCBOT : Gain  Gain=9.8056
  LCTOP : Gain  Gain=9.8056
  Mean : dspstat3/Mean  run=off  InputProcessing=Columns as channels (frame based)  reset_popup=None  directionMode=Each column  dimension=1  roiEnable=off  roiType=Rectangles  roiPortion=Entire ROI  roiOutput=Individual statistics for each ROI  roiFlag=off  roundingMode=Floor  overflowMode=off  outputDataTypeStr=Inherit: Same as accumulator  outputMin=[]  outputMax=[]  outputLastDataTypeStr=Inherit: Same as accumulator
  Mean1 : dspstat3/Mean  run=off  InputProcessing=Columns as channels (frame based)  reset_popup=None  directionMode=Each column  dimension=1  roiEnable=off  roiType=Rectangles  roiPortion=Entire ROI  roiOutput=Individual statistics for each ROI  roiFlag=off  roundingMode=Floor  overflowMode=off  outputDataTypeStr=Inherit: Same as accumulator  outputMin=[]  outputMax=[]  outputLastDataTypeStr=Inherit: Same as accumulator
  Switch : Switch  Criteria=u2 > Threshold  SaturateOnIntegerOverflow=off  InputSameDT=off
  Switch1 : Switch  Criteria=u2 > Threshold  SaturateOnIntegerOverflow=off  InputSameDT=off
  Zero : Constant  Value=0  OutDataTypeStr=Inherit: Inherit via back propagation
  Zero1 : Constant  Value=0  OutDataTypeStr=Inherit: Inherit via back propagation
  slope : Gain  Gain=1/1088.2909
  slope1 : Gain  Gain=1/857.4045
  zero offset : Constant  Value=4295.9625
  zero offset1 : Constant  Value=-6297.936
  tag scope: LCBotMass=global, LCTopMass=global, LCbot=global, LCbotRaw=global, LCtop=global, LCtopRaw=global
  wires:
  Byte Packing1/1 -> Mean1/1
  EtherCAT PDO Receive1/1 -> Byte Packing1/1
  Mean1/1 -> [LCbotRaw], Add1/1
  Byte Packing/1 -> Mean/1
  Switch/1 -> slope/1
  EtherCAT PDO Receive/1 -> Byte Packing/1
  slope/1 -> [LCTopMass], LCTOP/1  "LCtop_kg"
  LCTOP/1 -> [LCtop]  "lctop_N"
  LCBOT/1 -> [LCbot]  "lcbot_N"
  slope1/1 -> [LCBotMass], LCBOT/1  "LCbot_kg"
  Add1/1 -> Switch1/1
  zero offset1/1 -> Add1/2
  Zero/1 -> Switch/3
  [opState] -> Switch/2
  [opState] -> Switch1/2
  Zero1/1 -> Switch1/3
  Switch1/1 -> slope1/1
  Mean/1 -> [LCtopRaw], Add/1
  Add/1 -> Switch/1
  zero offset/1 -> Add/2

== system LUPAold/LUPAInputs/zero start ==
  pos_drv_rad : Inport
  Switch : Switch  Criteria=u2 > Threshold  SaturateOnIntegerOverflow=off  InputSameDT=off
  Zero : Constant  Value=0  OutDataTypeStr=double
  pos_rad_raw : Outport
  wires:
  [opState] -> Switch/2
  Switch/1 -> pos_rad_raw/1
  pos_drv_rad/1 -> Switch/1
  Zero/1 -> Switch/3

== matlab function LUPAold/Control/MATLAB Function ==
  data: controllerType input; x input; I_ctrl output; manualGains input; stiffness_Nperm output; time input; GainTstep input; ExcelGains input; Kt input; sprocketPitchRadius input; damping_Npermpers output
function [I_ctrl, stiffness_Nperm, damping_Npermpers] = fcn(controllerType, x, manualGains,time,GainTstep,ExcelGains, Kt, sprocketPitchRadius)
% gain format [positionProportional, velocityProportional]
% x format [theta; omega]

I_ctrl = 0;
gainMat = zeros(1,2);

if controllerType == 1

    B = sprocketPitchRadius^2 / Kt * manualGains' * x;
    stiffness_Nperm = manualGains(1);
    damping_Npermpers = manualGains(2);
elseif controllerType == 2
    idx = ceil(time./GainTstep); % Find index of current gain step
    while idx > length(ExcelGains(:,1))
        idx = idx-length(ExcelGains(:,1));
    end
    gainMat(1,1) = ExcelGains(idx,1);
    gainMat(1,2) = ExcelGains(idx,2);
    B = sprocketPitchRadius^2 / Kt * gainMat* x;
    stiffness_Nperm = gainMat(1,1);
    damping_Npermpers = gainMat(1,2);
else
    B = 0;
    stiffness_Nperm = 0;
    damping_Npermpers = 0;
end

I_ctrl = B;

== matlab function LUPAold/Initialization/controlword ==
  data: enabled input; clearfault input; statusword input; controlword output
function controlword = fcn(enabled, clearfault, statusword)

bitstatus = bitget(statusword,1:16);

if ~clearfault
    if enabled
        if bitstatus(1) == 0 % Ready to switch on not ready
            controlword = 6; % command ready switch on
        elseif ~bitstatus(2) % switched not yet on
            controlword = 7; % command switch on
        elseif ~bitstatus(3) % operation not yet enabled
            controlword = 15; % command enable
        else
            controlword = 15; % maintain enabled state
        end
    else
        controlword = 4; % command disabled
    end
else
    controlword = 128; % command clear faults
end
